simulink model "test_10gbe_out"  (Simulink 6.2)
settings: Solver=ode45  StartTime=0.0  StopTime=40000  RelTol=1e-3
libraries: xbsIndex_r3 x217, casper_library x8, xps_library x5
(part 1 of 2)
settings Model: LastModifiedBy=Jason Manley
settings DebuggingCC: SolverPrmCheckMsg=warning

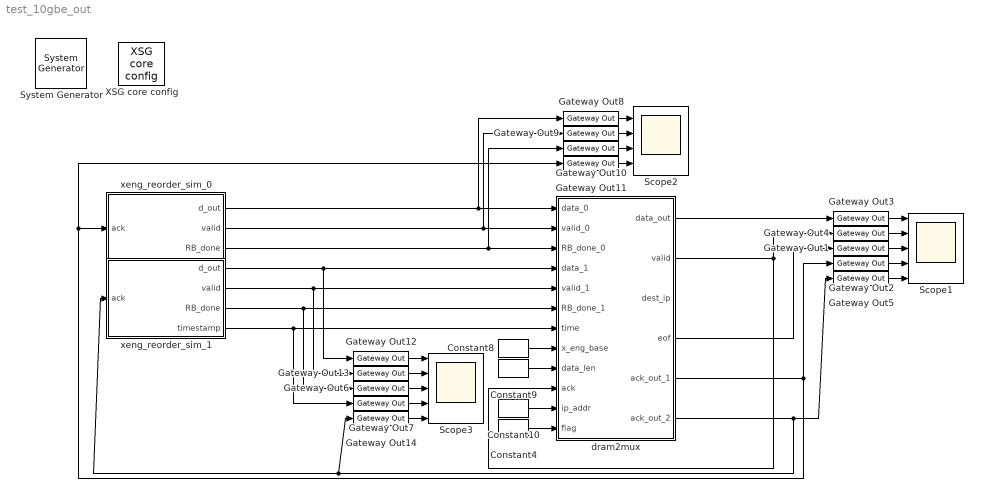
== system test_10gbe_out ==
  " System Generator" : xbsIndex_r3/ System Generator  Tag=genX  xilinxfamily=Virtex2  part=xc2v1000  speed=-4  package=bg575  synthesis_tool=XST  directory=./netlist  testbench=off  simulink_period=1  sysclk_period=100  incr_netlist=off  trim_vbits=Everywhere in SubSystem  dbl_ovrd=According to Block Masks  core_generation=According to Block Masks  run_coregen=off  deprecated_control=off  eval_field=0
      settings: AttributesFormatString=System\nGenerator
  Constant10 : xbsIndex_r3/Constant  const=1000  equ=P=C  arith_type=Unsigned  n_bits=32  bin_pt=0  opselect=C  inp2=PCIN>>17  opr=+  inp1=P  carry=CIN  iostate=0  explicit_period=on  period=1  dbl_ovrd=off
  Constant4 : xbsIndex_r3/Constant  const=0  equ=P=C  arith_type=Unsigned  n_bits=32  bin_pt=0  opselect=C  inp2=PCIN>>17  opr=+  inp1=P  carry=CIN  iostate=0  explicit_period=on  period=1  dbl_ovrd=off
  Constant8 : xbsIndex_r3/Constant  const=8  equ=P=C  arith_type=Unsigned  n_bits=16  bin_pt=0  opselect=C  inp2=PCIN>>17  opr=+  inp1=P  carry=CIN  iostate=0  explicit_period=on  period=1  dbl_ovrd=off
  Constant9 : xbsIndex_r3/Constant  const=180  equ=P=C  arith_type=Unsigned  n_bits=32  bin_pt=0  opselect=C  inp2=PCIN>>17  opr=+  inp1=P  carry=CIN  iostate=0  explicit_period=on  period=1  dbl_ovrd=off
  Gateway Out{1..14} (14 alike) : xbsIndex_r3/Gateway Out  output_type=Double  nbits=8  bin_pt=6  arith_type=Boolean  quantization=Truncate  overflow=Wrap  hdl_port=on  timing_constraint=None  locs_specified=off  LOCs={}  needs_fixed_name=off  show_param=off
      settings: xl_area=[0, 0, 0, 0, 0, 0, 0]
  Scope1 : Scope  NumInputPorts=5
      settings: YMin=432~-1~-1~-1~0  YMax=432~1~1~1~1  SaveName=ScopeData2
  Scope2 : Scope  NumInputPorts=4
      settings: YMin=0~0.95~0.95~-1  YMax=1~1.05~1.05~1
  Scope3 : Scope  NumInputPorts=5
      settings: YMin=10600~1~-1~-1~0  YMax=12200~1~1~1~1
  XSG core config : xps_library/XSG core config  Tag=xps:xsg  hw_sys=BEE2_usr  ibob_linux=off  clk_src=sys_clk2x  gpio_clk_io_group=iBOB:sma  gpio_clk_bit_index=0  clk_rate=205  sample_period=1  synthesis_tool=XST  mpc_type=powerpc405
  dram2mux : Subsystem  mask{payload_len=180}
      mask prompts: payload_len "Payload length"
  xeng_reorder_sim_0 : Subsystem
  xeng_reorder_sim_1 : Subsystem
  wires:
  dram2mux/5(ack_out_1) -> Gateway Out2/1, Gateway Out11/1, xeng_reorder_sim_0/1(ack)
  dram2mux/6(ack_out_2) -> Gateway Out5/1, Gateway Out14/1, xeng_reorder_sim_1/1(ack)
  Constant4/1 -> dram2mux/12(flag)
  Constant9/1 -> dram2mux/9(data_len)
  Constant10/1 -> dram2mux/11(ip_addr)
  dram2mux/2(valid) -> dram2mux/10(ack), Gateway Out4/1
  Gateway Out8/1 -> Scope2/1
  Gateway Out9/1 -> Scope2/2
  Gateway Out10/1 -> Scope2/3
  Gateway Out11/1 -> Scope2/4
  Gateway Out3/1 -> Scope1/1
  Gateway Out4/1 -> Scope1/2
  Gateway Out1/1 -> Scope1/3
  Gateway Out2/1 -> Scope1/4
  dram2mux/1(data_out) -> Gateway Out3/1
  dram2mux/4(eof) -> Gateway Out1/1
  Gateway Out5/1 -> Scope1/5
  xeng_reorder_sim_0/1(d_out) -> dram2mux/1(data_0), Gateway Out8/1
  xeng_reorder_sim_0/2(valid) -> dram2mux/2(valid_0), Gateway Out9/1
  Constant8/1 -> dram2mux/8(x_eng_base)
  xeng_reorder_sim_0/3(RB_done) -> dram2mux/3(RB_done_0), Gateway Out10/1
  xeng_reorder_sim_1/1(d_out) -> dram2mux/4(data_1), Gateway Out12/1
  xeng_reorder_sim_1/2(valid) -> dram2mux/5(valid_1), Gateway Out13/1
  xeng_reorder_sim_1/3(RB_done) -> dram2mux/6(RB_done_1), Gateway Out6/1
  xeng_reorder_sim_1/4(timestamp) -> dram2mux/7(time), Gateway Out7/1
  Gateway Out12/1 -> Scope3/1
  Gateway Out13/1 -> Scope3/2
  Gateway Out6/1 -> Scope3/3
  Gateway Out7/1 -> Scope3/4
  Gateway Out14/1 -> Scope3/5

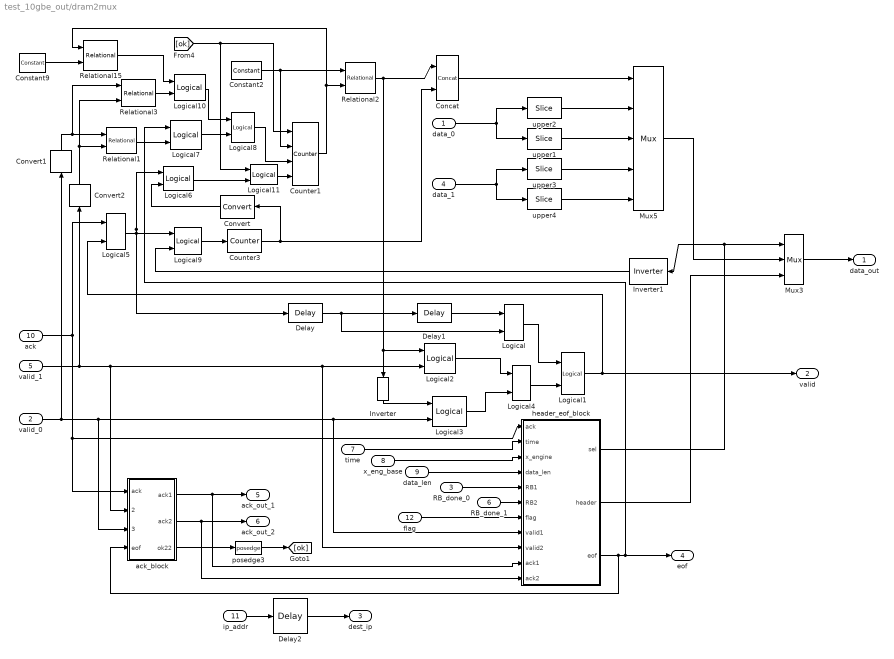
== system test_10gbe_out/dram2mux ==
  data_0 : Inport  Port=1  LatchInput=off
  valid_0 : Inport  Port=2  LatchInput=off
  RB_done_0 : Inport  Port=3  LatchInput=off
  data_1 : Inport  Port=4  LatchInput=off
  valid_1 : Inport  Port=5  LatchInput=off
  RB_done_1 : Inport  Port=6  LatchInput=off
  time : Inport  Port=7  LatchInput=off
  x_eng_base : Inport  Port=8  LatchInput=off
  data_len : Inport  Port=9  LatchInput=off
  ack : Inport  Port=10  LatchInput=off
  ip_addr : Inport  Port=11  LatchInput=off
  flag : Inport  Port=12  LatchInput=off
  Concat : xbsIndex_r3/Concat  num_inputs=2  explicit_period=off  period=1  dbl_ovrd=off
  Constant2 : xbsIndex_r3/Constant  const=payload_len/2  equ=P=C  arith_type=Unsigned  n_bits=16  bin_pt=0  opselect=C  inp2=PCIN>>17  opr=+  inp1=P  carry=CIN  iostate=0  explicit_period=on  period=1  dbl_ovrd=off
  Constant9 : xbsIndex_r3/Constant  const=payload_len  equ=P=C  arith_type=Unsigned  n_bits=8  bin_pt=0  opselect=C  inp2=PCIN>>17  opr=+  inp1=P  carry=CIN  iostate=0  explicit_period=on  period=1  dbl_ovrd=off
  Convert : xbsIndex_r3/Convert  Orientation=left  arith_type=Boolean  n_bits=8  bin_pt=6  quantization=Truncate  overflow=Wrap  latency=0  explicit_period=off  period=1  dbl_ovrd=off  show_param=off  inserted_by_tool=off  pipeline=off
      settings: xl_area=[0, 0, 0, 0, 0, 0, 0]
  Convert1 : xbsIndex_r3/Convert  Orientation=up  arith_type=Unsigned  n_bits=1  bin_pt=0  quantization=Truncate  overflow=Wrap  latency=0  explicit_period=off  period=1  dbl_ovrd=off  show_param=off  inserted_by_tool=off  pipeline=off
      settings: xl_area=[0, 0, 0, 0, 0, 0, 0]
  Convert2 : xbsIndex_r3/Convert  Orientation=up  arith_type=Unsigned  n_bits=1  bin_pt=0  quantization=Truncate  overflow=Wrap  latency=0  explicit_period=off  period=1  dbl_ovrd=off  show_param=off  inserted_by_tool=off  pipeline=off
      settings: xl_area=[0, 0, 0, 0, 0, 0, 0]
  Counter1 : xbsIndex_r3/Counter  cnt_type=Free Running  n_bits=16  bin_pt=0  arith_type=Unsigned  start_count=0  cnt_to=180  cnt_by_val=1  operation=Up  explicit_period=on  period=1  load_pin=on  rst=on  en=on  dbl_ovrd=off  show_param=off  use_rpm=on  gen_core=off
      settings: xl_area=[0, 0, 0, 0, 0, 0, 0]
  Counter3 : xbsIndex_r3/Counter  cnt_type=Free Running  n_bits=1  bin_pt=0  arith_type=Unsigned  start_count=0  cnt_to=Inf  cnt_by_val=1  operation=Up  explicit_period=on  period=1  load_pin=off  rst=off  en=on  dbl_ovrd=off  show_param=off  use_rpm=on  gen_core=off
      settings: xl_area=[0, 0, 0, 0, 0, 0, 0]
  Delay : xbsIndex_r3/Delay  latency=1  reg_retiming=off  explicit_period=on  period=1  en=off  accept_only_valid=off  init_zero=on  dbl_ovrd=off  show_param=off
      settings: xl_area=[0, 0, 0, 0, 0, 0, 0]
  Delay1 : xbsIndex_r3/Delay  latency=1  reg_retiming=off  explicit_period=on  period=1  en=off  accept_only_valid=off  init_zero=on  dbl_ovrd=off  show_param=off
      settings: xl_area=[0, 0, 0, 0, 0, 0, 0]
  Delay2 : xbsIndex_r3/Delay  latency=2  reg_retiming=off  explicit_period=off  period=1  en=off  accept_only_valid=off  init_zero=on  dbl_ovrd=off  show_param=off
      settings: xl_area=[0, 0, 0, 0, 0, 0, 0]
  Inverter : xbsIndex_r3/Inverter  Orientation=down  latency=0  explicit_period=off  period=1  en=off  dbl_ovrd=off  show_param=off
      settings: xl_area=[0, 0, 0, 0, 0, 0, 0]
  Inverter1 : xbsIndex_r3/Inverter  Orientation=left  latency=0  explicit_period=off  period=1  en=off  dbl_ovrd=off  show_param=off
      settings: xl_area=[0, 0, 0, 0, 0, 0, 0]
  Logical : xbsIndex_r3/Logical  logical_function=NOR  inputs=2  precision=Full  arith_type=Unsigned  n_bits=8  bin_pt=2  align_bp=on  latency=0  explicit_period=off  period=1  en=off  dbl_ovrd=off  show_param=off
      settings: xl_area=[0, 0, 0, 0, 0, 0, 0]
  Logical{1..3,5..7,10} (7 alike) : xbsIndex_r3/Logical  logical_function=AND  inputs=2  precision=Full  arith_type=Unsigned  n_bits=8  bin_pt=2  align_bp=off  latency=0  explicit_period=off  period=1  en=off  dbl_ovrd=off  show_param=off
      settings: xl_area=[0, 0, 0, 0, 0, 0, 0]
  Logical11 : xbsIndex_r3/Logical  logical_function=OR  inputs=2  precision=Full  arith_type=Unsigned  n_bits=8  bin_pt=2  align_bp=off  latency=0  explicit_period=off  period=1  en=off  dbl_ovrd=off  show_param=off
      settings: xl_area=[0, 0, 0, 0, 0, 0, 0]
  Logical4 : xbsIndex_r3/Logical  logical_function=OR  inputs=2  precision=Full  arith_type=Unsigned  n_bits=8  bin_pt=2  align_bp=on  latency=2  explicit_period=off  period=1  en=off  dbl_ovrd=off  show_param=off
      settings: xl_area=[0, 0, 0, 0, 0, 0, 0]
  Logical8 : xbsIndex_r3/Logical  logical_function=OR  inputs=2  precision=Full  arith_type=Unsigned  n_bits=8  bin_pt=2  align_bp=off  latency=0  explicit_period=off  period=1  en=off  dbl_ovrd=off  show_param=off
      settings: xl_area=[0, 0, 0, 0, 0, 0, 0]
  Logical9 : xbsIndex_r3/Logical  logical_function=AND  inputs=2  precision=Full  arith_type=Unsigned  n_bits=8  bin_pt=2  align_bp=on  latency=0  explicit_period=off  period=1  en=off  dbl_ovrd=off  show_param=off
      settings: xl_area=[0, 0, 0, 0, 0, 0, 0]
  Mux3 : xbsIndex_r3/Mux  inputs=2  precision=Full  arith_type="Signed  (2's comp)"  n_bits=8  bin_pt=2  quantization=Truncate  overflow=Wrap  latency=0  explicit_period=off  period=1  en=off  dbl_ovrd=off  show_param=off  mux_type=off  use_rpm=off  gen_core=off
      settings: xl_area=[0, 0, 0, 0, 0, 0, 0]
  Mux5 : xbsIndex_r3/Mux  inputs=4  precision=Full  arith_type="Signed  (2's comp)"  n_bits=8  bin_pt=2  quantization=Truncate  overflow=Wrap  latency=2  explicit_period=on  period=1  en=off  dbl_ovrd=off  show_param=off  mux_type=off  use_rpm=off  gen_core=off
      settings: xl_area=[0, 0, 0, 0, 0, 0, 0]
  Relational1 : xbsIndex_r3/Relational  mode=a>b  latency=0  explicit_period=off  period=1  en=off  dbl_ovrd=off  show_param=off
      settings: xl_area=[0, 0, 0, 0, 0, 0, 0]
  Relational15 : xbsIndex_r3/Relational  mode=a=b  latency=1  explicit_period=off  period=1  en=off  dbl_ovrd=off  show_param=off
      settings: xl_area=[0, 0, 0, 0, 0, 0, 0]
  Relational2 : xbsIndex_r3/Relational  mode=a<=b  latency=0  explicit_period=off  period=1  en=off  dbl_ovrd=off  show_param=off
      settings: xl_area=[0, 0, 0, 0, 0, 0, 0]
  Relational3 : xbsIndex_r3/Relational  mode=a>b  latency=0  explicit_period=off  period=1  en=off  dbl_ovrd=off  show_param=off
      settings: xl_area=[0, 0, 0, 0, 0, 0, 0]
  ack_block : Subsystem
  header_eof_block : Subsystem
  posedge3 : casper_library/Misc/posedge  Tag=Rising Edge Detector
  upper1 : xbsIndex_r3/Slice  mode=Lower Bit Location + Width  nbits=64  bit1=0  base1=MSB of Input  bit0=0  base0=LSB of Input  boolean_output=off  explicit_period=off  period=1  dbl_ovrd=off
  upper2 : xbsIndex_r3/Slice  mode=Upper Bit Location + Width  nbits=64  bit1=0  base1=MSB of Input  bit0=0  base0=LSB of Input  boolean_output=off  explicit_period=off  period=1  dbl_ovrd=off
  upper3 : xbsIndex_r3/Slice  mode=Upper Bit Location + Width  nbits=64  bit1=0  base1=MSB of Input  bit0=0  base0=LSB of Input  boolean_output=off  explicit_period=off  period=1  dbl_ovrd=off
  upper4 : xbsIndex_r3/Slice  mode=Lower Bit Location + Width  nbits=64  bit1=0  base1=MSB of Input  bit0=0  base0=LSB of Input  boolean_output=off  explicit_period=off  period=1  dbl_ovrd=off
  data_out : Outport
  valid : Outport  Port=2
  dest_ip : Outport  Port=3
  eof : Outport  Port=4
  ack_out_1 : Outport  Port=5
  ack_out_2 : Outport  Port=6
  wires:
  ack_block/2(ack2) -> ack_out_2/1, header_eof_block/11(ack2)
  ack_block/1(ack1) -> ack_out_1/1, header_eof_block/10(ack1)
  Inverter1/1 -> Logical9/2
  Mux5/1 -> Mux3/2
  data_len/1 -> header_eof_block/4(data_len)
  Delay2/1 -> dest_ip/1
  ip_addr/1 -> Delay2/1
  Mux3/1 -> data_out/1
  header_eof_block/2(header) -> Mux3/3
  x_eng_base/1 -> header_eof_block/3(x_engine)
  time/1 -> header_eof_block/2(time)
  Logical5/1 -> Logical6/1, Logical9/1, Delay/1
  Logical4/1 -> Logical1/2
  Logical3/1 -> Logical4/2
  Logical2/1 -> Logical4/1
  valid_1/1 -> ack_block/2(valid2), Logical2/2, header_eof_block/9(valid2), Convert2/1
  valid_0/1 -> ack_block/3(valid1), Logical3/2, header_eof_block/8(valid1), Convert1/1
  Logical1/1 -> valid/1, Logical5/2
  Logical/1 -> Logical1/1
  Delay1/1 -> Logical/1
  Delay/1 -> Delay1/1, Logical/2
  ack/1 -> Logical5/1, header_eof_block/1(ack), ack_block/1(ack)
  Concat/1 -> Mux5/1
  Relational2/1 -> Inverter/1, Logical2/1, Concat/1
  Constant2/1 -> Relational2/1, Counter1/2
  data_1/1 -> upper3/1, upper4/1
  data_0/1 -> upper2/1, upper1/1
  upper4/1 -> Mux5/5
  upper3/1 -> Mux5/4
  upper1/1 -> Mux5/3
  upper2/1 -> Mux5/2
  Inverter/1 -> Logical3/1
  Convert/1 -> Logical6/2
  Counter3/1 -> Convert/1, Concat/2
  Logical9/1 -> Counter3/1
  Constant9/1 -> Relational15/2
  header_eof_block/1(sel) -> Inverter1/1, Mux3/1
  header_eof_block/3(eof) -> eof/1, Logical7/1, ack_block/4(eof)
  RB_done_0/1 -> header_eof_block/5(RB1)
  RB_done_1/1 -> header_eof_block/6(RB2)
  flag/1 -> header_eof_block/7(flag)
  Logical7/1 -> Logical8/2
  Relational1/1 -> Logical7/2
  Convert1/1 -> Relational1/1, Relational3/1
  Convert2/1 -> Relational1/2, Relational3/2
  Relational15/1 -> Logical10/1
  Relational3/1 -> Logical10/2
  Logical8/1 -> Counter1/3
  Logical6/1 -> Logical11/2
  Logical11/1 -> Counter1/4
  ack_block/3(ok22) -> posedge3/1
  posedge3/1 -> [ok]
  Logical10/1 -> Logical8/1
  Counter1/1 -> Relational2/2, Relational15/1
  [ok] -> Counter1/1, Logical11/1

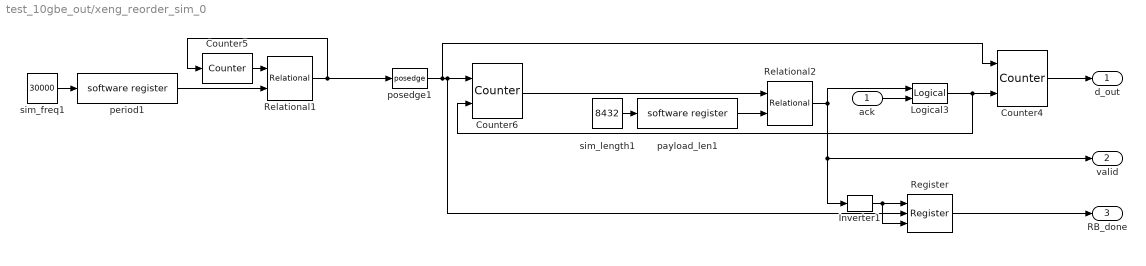
== system test_10gbe_out/xeng_reorder_sim_0 ==
  ack : Inport  Port=1  LatchInput=off
  Counter4 : xbsIndex_r3/Counter  cnt_type=Free Running  n_bits=64  bin_pt=0  arith_type=Unsigned  start_count=0  cnt_to=Inf  cnt_by_val=1  operation=Up  explicit_period=off  period=1  load_pin=off  rst=on  en=on  dbl_ovrd=off  show_param=off  use_rpm=off  gen_core=off
      settings: xl_area=[0, 0, 0, 0, 0, 0, 0]
  Counter5 : xbsIndex_r3/Counter  cnt_type=Free Running  n_bits=32  bin_pt=0  arith_type=Unsigned  start_count=1  cnt_to=Inf  cnt_by_val=1  operation=Up  explicit_period=on  period=1  load_pin=off  rst=on  en=off  dbl_ovrd=off  show_param=off  use_rpm=on  gen_core=off
      settings: xl_area=[0, 0, 0, 0, 0, 0, 0]
  Counter6 : xbsIndex_r3/Counter  cnt_type=Free Running  n_bits=32  bin_pt=0  arith_type=Unsigned  start_count=0  cnt_to=1023  cnt_by_val=1  operation=Up  explicit_period=on  period=1  load_pin=off  rst=on  en=on  dbl_ovrd=off  show_param=off  use_rpm=on  gen_core=off
      settings: xl_area=[0, 0, 0, 0, 0, 0, 0]
  Inverter1 : xbsIndex_r3/Inverter  latency=0  explicit_period=off  period=1  en=off  dbl_ovrd=off  show_param=off
      settings: xl_area=[0, 0, 0, 0, 0, 0, 0]
  Logical3 : xbsIndex_r3/Logical  logical_function=AND  inputs=2  precision=Full  arith_type=Unsigned  n_bits=8  bin_pt=2  align_bp=on  latency=0  explicit_period=off  period=1  en=off  dbl_ovrd=off  show_param=off
      settings: xl_area=[0, 0, 0, 0, 0, 0, 0]
  Register : xbsIndex_r3/Register  init=0  reg_only_valid=off  explicit_period=off  period=1  rst=on  en=on  out_en=off  dbl_ovrd=off  show_param=off
      settings: xl_area=[0, 0, 0, 0, 0, 0, 0]
  Relational1 : xbsIndex_r3/Relational  mode=a>=b  latency=0  explicit_period=on  period=1  en=off  dbl_ovrd=off  show_param=off
      settings: xl_area=[0, 0, 0, 0, 0, 0, 0]
  Relational2 : xbsIndex_r3/Relational  mode=a<b  latency=0  explicit_period=off  period=1  en=off  dbl_ovrd=off  show_param=off
      settings: xl_area=[0, 0, 0, 0, 0, 0, 0]
  payload_len1 : xps_library/software register  Tag=xps:sw_reg  io_dir=From Processor  arith_type=Unsigned  bitwidth=32  bin_pt=0  sample_period=1  gw_name=test_10gbe_out_xeng_reorder_sim_0_payload_len1_user_data_out
  period1 : xps_library/software register  Tag=xps:sw_reg  io_dir=From Processor  arith_type=Unsigned  bitwidth=32  bin_pt=0  sample_period=1  gw_name=test_10gbe_out_xeng_reorder_sim_0_period1_user_data_out
  posedge1 : casper_library/Misc/pulse_ext/posedge  Tag=Rising Edge Detector
  sim_freq1 : Constant  Value=30000
  sim_length1 : Constant  Value=8432
  d_out : Outport
  valid : Outport  Port=2
  RB_done : Outport  Port=3
  wires:
  Counter5/1 -> Relational1/1
  Relational1/1 -> Counter5/1, posedge1/1
  Counter4/1 -> d_out/1
  period1/1 -> Relational1/2
  sim_freq1/1 -> period1/1
  Relational2/1 -> Inverter1/1, valid/1, Logical3/1
  Counter6/1 -> Relational2/1
  posedge1/1 -> Counter4/1, Counter6/1, Register/2
  sim_length1/1 -> payload_len1/1
  Logical3/1 -> Counter4/2, Counter6/2
  payload_len1/1 -> Relational2/2
  Register/1 -> RB_done/1
  Inverter1/1 -> Register/1, Register/3
  ack/1 -> Logical3/2

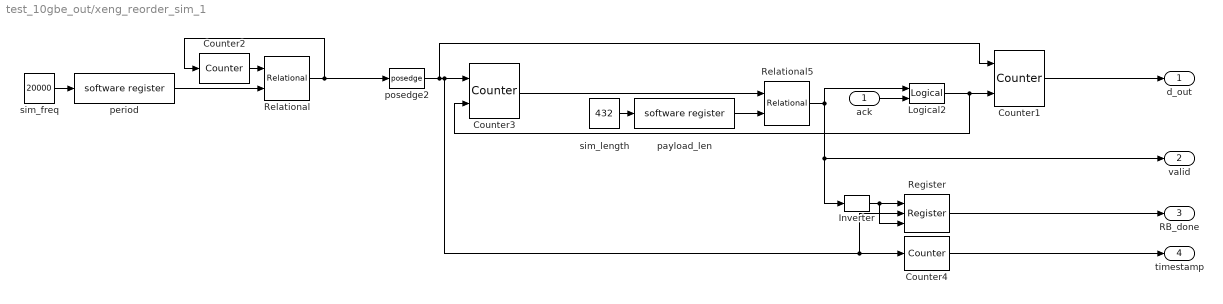
== system test_10gbe_out/xeng_reorder_sim_1 ==
  ack : Inport  Port=1  LatchInput=off
  Counter1 : xbsIndex_r3/Counter  cnt_type=Free Running  n_bits=64  bin_pt=0  arith_type=Unsigned  start_count=0  cnt_to=Inf  cnt_by_val=1  operation=Up  explicit_period=off  period=1  load_pin=off  rst=on  en=on  dbl_ovrd=off  show_param=off  use_rpm=off  gen_core=off
      settings: xl_area=[0, 0, 0, 0, 0, 0, 0]
  Counter2 : xbsIndex_r3/Counter  cnt_type=Free Running  n_bits=32  bin_pt=0  arith_type=Unsigned  start_count=1  cnt_to=Inf  cnt_by_val=1  operation=Up  explicit_period=on  period=1  load_pin=off  rst=on  en=off  dbl_ovrd=off  show_param=off  use_rpm=on  gen_core=off
      settings: xl_area=[0, 0, 0, 0, 0, 0, 0]
  Counter3 : xbsIndex_r3/Counter  cnt_type=Free Running  n_bits=32  bin_pt=0  arith_type=Unsigned  start_count=0  cnt_to=1023  cnt_by_val=1  operation=Up  explicit_period=on  period=1  load_pin=off  rst=on  en=on  dbl_ovrd=off  show_param=off  use_rpm=on  gen_core=off
      settings: xl_area=[0, 0, 0, 0, 0, 0, 0]
  Counter4 : xbsIndex_r3/Counter  cnt_type=Free Running  n_bits=64  bin_pt=0  arith_type=Unsigned  start_count=0  cnt_to=1023  cnt_by_val=1  operation=Up  explicit_period=on  period=1  load_pin=off  rst=off  en=on  dbl_ovrd=off  show_param=off  use_rpm=on  gen_core=off
      settings: xl_area=[0, 0, 0, 0, 0, 0, 0]
  Inverter : xbsIndex_r3/Inverter  latency=0  explicit_period=off  period=1  en=off  dbl_ovrd=off  show_param=off
      settings: xl_area=[0, 0, 0, 0, 0, 0, 0]
  Logical2 : xbsIndex_r3/Logical  logical_function=AND  inputs=2  precision=Full  arith_type=Unsigned  n_bits=8  bin_pt=2  align_bp=on  latency=0  explicit_period=off  period=1  en=off  dbl_ovrd=off  show_param=off
      settings: xl_area=[0, 0, 0, 0, 0, 0, 0]
  Register : xbsIndex_r3/Register  init=0  reg_only_valid=off  explicit_period=off  period=1  rst=on  en=on  out_en=off  dbl_ovrd=off  show_param=off
      settings: xl_area=[0, 0, 0, 0, 0, 0, 0]
  Relational : xbsIndex_r3/Relational  mode=a>=b  latency=0  explicit_period=on  period=1  en=off  dbl_ovrd=off  show_param=off
      settings: xl_area=[0, 0, 0, 0, 0, 0, 0]
  Relational5 : xbsIndex_r3/Relational  mode=a<b  latency=0  explicit_period=off  period=1  en=off  dbl_ovrd=off  show_param=off
      settings: xl_area=[0, 0, 0, 0, 0, 0, 0]
  payload_len : xps_library/software register  Tag=xps:sw_reg  io_dir=From Processor  arith_type=Unsigned  bitwidth=32  bin_pt=0  sample_period=1  gw_name=test_10gbe_out_xeng_reorder_sim_1_payload_len_user_data_out
  period : xps_library/software register  Tag=xps:sw_reg  io_dir=From Processor  arith_type=Unsigned  bitwidth=32  bin_pt=0  sample_period=1  gw_name=test_10gbe_out_xeng_reorder_sim_1_period_user_data_out
  posedge2 : casper_library/Misc/pulse_ext/posedge  Tag=Rising Edge Detector
  sim_freq : Constant  Value=20000
  sim_length : Constant  Value=432
  d_out : Outport
  valid : Outport  Port=2
  RB_done : Outport  Port=3
  timestamp : Outport  Port=4
  wires:
  Counter2/1 -> Relational/1
  Relational/1 -> Counter2/1, posedge2/1
  Counter1/1 -> d_out/1
  period/1 -> Relational/2
  sim_freq/1 -> period/1
  Relational5/1 -> Inverter/1, valid/1, Logical2/1
  Counter3/1 -> Relational5/1
  posedge2/1 -> Counter1/1, Counter3/1, Counter4/1, Register/2
  sim_length/1 -> payload_len/1
  Logical2/1 -> Counter1/2, Counter3/2
  payload_len/1 -> Relational5/2
  Register/1 -> RB_done/1
  Counter4/1 -> timestamp/1
  Inverter/1 -> Register/1, Register/3
  ack/1 -> Logical2/2

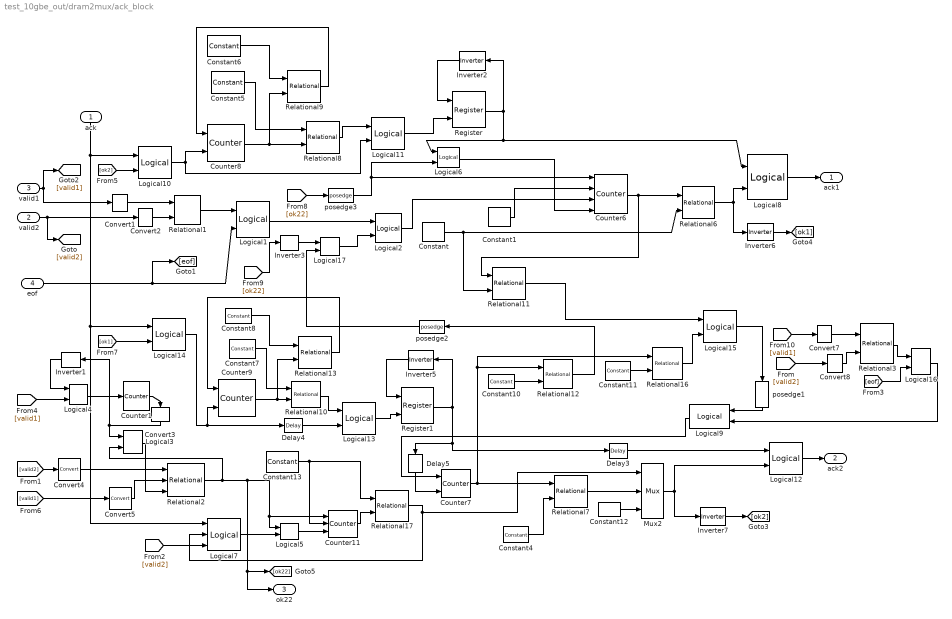
== system test_10gbe_out/dram2mux/ack_block ==
  ack : Inport  Orientation=down  Port=1  LatchInput=off
  valid2 : Inport  Port=2  LatchInput=off
  valid1 : Inport  Port=3  LatchInput=off
  eof : Inport  Port=4  LatchInput=off
  Constant : xbsIndex_r3/Constant  const=payload_len*3/2 -1  equ=P=C  arith_type=Unsigned  n_bits=10  bin_pt=0  opselect=C  inp2=PCIN>>17  opr=+  inp1=P  carry=CIN  iostate=0  explicit_period=on  period=1  dbl_ovrd=off
  Constant1 : xbsIndex_r3/Constant  const=payload_len*3/2  equ=P=C  arith_type=Unsigned  n_bits=10  bin_pt=0  opselect=C  inp2=PCIN>>17  opr=+  inp1=P  carry=CIN  iostate=0  explicit_period=on  period=1  dbl_ovrd=off
  Constant10 : xbsIndex_r3/Constant  const=payload_len*3/2 -1  equ=P=C  arith_type=Unsigned  n_bits=9  bin_pt=0  opselect=C  inp2=PCIN>>17  opr=+  inp1=P  carry=CIN  iostate=0  explicit_period=on  period=1  dbl_ovrd=off
  Constant11 : xbsIndex_r3/Constant  const=payload_len*3/2+1  equ=P=C  arith_type=Unsigned  n_bits=9  bin_pt=0  opselect=C  inp2=PCIN>>17  opr=+  inp1=P  carry=CIN  iostate=0  explicit_period=on  period=1  dbl_ovrd=off
  Constant12 : xbsIndex_r3/Constant  const=0  equ=P=C  arith_type=Boolean  n_bits=1  bin_pt=0  opselect=C  inp2=PCIN>>17  opr=+  inp1=P  carry=CIN  iostate=0  explicit_period=on  period=1  dbl_ovrd=off
  Constant13 : xbsIndex_r3/Constant  const=payload_len+3  equ=P=C  arith_type=Unsigned  n_bits=10  bin_pt=0  opselect=C  inp2=PCIN>>17  opr=+  inp1=P  carry=CIN  iostate=0  explicit_period=on  period=1  dbl_ovrd=off
  Constant4 : xbsIndex_r3/Constant  const=payload_len*3/2-1  equ=P=C  arith_type=Unsigned  n_bits=9  bin_pt=0  opselect=C  inp2=PCIN>>17  opr=+  inp1=P  carry=CIN  iostate=0  explicit_period=on  period=1  dbl_ovrd=off
  Constant5 : xbsIndex_r3/Constant  const=3  equ=P=C  arith_type=Unsigned  n_bits=2  bin_pt=0  opselect=C  inp2=PCIN>>17  opr=+  inp1=P  carry=CIN  iostate=0  explicit_period=on  period=1  dbl_ovrd=off
  Constant6 : xbsIndex_r3/Constant  const=payload_len+3  equ=P=C  arith_type=Unsigned  n_bits=8  bin_pt=0  opselect=C  inp2=PCIN>>17  opr=+  inp1=P  carry=CIN  iostate=0  explicit_period=on  period=1  dbl_ovrd=off
  Constant7 : xbsIndex_r3/Constant  const=3  equ=P=C  arith_type=Unsigned  n_bits=2  bin_pt=0  opselect=C  inp2=PCIN>>17  opr=+  inp1=P  carry=CIN  iostate=0  explicit_period=on  period=1  dbl_ovrd=off
  Constant8 : xbsIndex_r3/Constant  const=payload_len+3  equ=P=C  arith_type=Unsigned  n_bits=8  bin_pt=0  opselect=C  inp2=PCIN>>17  opr=+  inp1=P  carry=CIN  iostate=0  explicit_period=on  period=1  dbl_ovrd=off
  Convert{1..2,4..5,7..8} (6 alike) : xbsIndex_r3/Convert  arith_type=Unsigned  n_bits=1  bin_pt=0  quantization=Truncate  overflow=Wrap  latency=0  explicit_period=off  period=1  dbl_ovrd=off  show_param=off  inserted_by_tool=off  pipeline=off
      settings: xl_area=[0, 0, 0, 0, 0, 0, 0]
  Convert3 : xbsIndex_r3/Convert  Orientation=down  arith_type=Boolean  n_bits=1  bin_pt=0  quantization=Truncate  overflow=Wrap  latency=0  explicit_period=off  period=1  dbl_ovrd=off  show_param=off  inserted_by_tool=off  pipeline=off
      settings: xl_area=[0, 0, 0, 0, 0, 0, 0]
  Counter1 : xbsIndex_r3/Counter  cnt_type=Count Limited  n_bits=1  bin_pt=0  arith_type=Unsigned  start_count=0  cnt_to=1  cnt_by_val=1  operation=Up  explicit_period=on  period=1  load_pin=off  rst=off  en=on  dbl_ovrd=off  show_param=off  use_rpm=on  gen_core=off
      settings: xl_area=[0, 0, 0, 0, 0, 0, 0]
  Counter11 : xbsIndex_r3/Counter  cnt_type=Free Running  n_bits=10  bin_pt=0  arith_type=Unsigned  start_count=0  cnt_to=Inf  cnt_by_val=1  operation=Up  explicit_period=on  period=1  load_pin=on  rst=off  en=on  dbl_ovrd=off  show_param=off  use_rpm=on  gen_core=off
      settings: xl_area=[0, 0, 0, 0, 0, 0, 0]
  Counter6 : xbsIndex_r3/Counter  cnt_type=Free Running  n_bits=10  bin_pt=0  arith_type=Unsigned  start_count=0  cnt_to=Inf  cnt_by_val=1  operation=Up  explicit_period=on  period=1  load_pin=on  rst=on  en=on  dbl_ovrd=off  show_param=off  use_rpm=on  gen_core=off
      settings: xl_area=[0, 0, 0, 0, 0, 0, 0]
  Counter7 : xbsIndex_r3/Counter  cnt_type=Free Running  n_bits=10  bin_pt=0  arith_type=Unsigned  start_count=0  cnt_to=Inf  cnt_by_val=1  operation=Up  explicit_period=on  period=1  load_pin=off  rst=on  en=on  dbl_ovrd=off  show_param=off  use_rpm=on  gen_core=off
      settings: xl_area=[0, 0, 0, 0, 0, 0, 0]
  Counter8 : xbsIndex_r3/Counter  cnt_type=Free Running  n_bits=8  bin_pt=0  arith_type=Unsigned  start_count=0  cnt_to=Inf  cnt_by_val=1  operation=Up  explicit_period=on  period=1  load_pin=off  rst=on  en=on  dbl_ovrd=off  show_param=off  use_rpm=on  gen_core=off
      settings: xl_area=[0, 0, 0, 0, 0, 0, 0]
  Counter9 : xbsIndex_r3/Counter  cnt_type=Free Running  n_bits=8  bin_pt=0  arith_type=Unsigned  start_count=0  cnt_to=Inf  cnt_by_val=1  operation=Up  explicit_period=on  period=1  load_pin=off  rst=on  en=on  dbl_ovrd=off  show_param=off  use_rpm=on  gen_core=off
      settings: xl_area=[0, 0, 0, 0, 0, 0, 0]
  Delay3 : xbsIndex_r3/Delay  latency=1  reg_retiming=off  explicit_period=on  period=1  en=off  accept_only_valid=off  init_zero=on  dbl_ovrd=off  show_param=off
      settings: xl_area=[0, 0, 0, 0, 0, 0, 0]
  Delay4 : xbsIndex_r3/Delay  latency=2  reg_retiming=off  explicit_period=on  period=1  en=off  accept_only_valid=off  init_zero=on  dbl_ovrd=off  show_param=off
      settings: xl_area=[0, 0, 0, 0, 0, 0, 0]
  Delay5 : xbsIndex_r3/Delay  Orientation=down  latency=1  reg_retiming=off  explicit_period=on  period=1  en=off  accept_only_valid=off  init_zero=on  dbl_ovrd=off  show_param=off
      settings: xl_area=[0, 0, 0, 0, 0, 0, 0]
  Inverter1 : xbsIndex_r3/Inverter  Orientation=left  latency=0  explicit_period=off  period=1  en=off  dbl_ovrd=off  show_param=off
      settings: xl_area=[0, 0, 0, 0, 0, 0, 0]
  Inverter2 : xbsIndex_r3/Inverter  Orientation=left  latency=0  explicit_period=off  period=1  en=off  dbl_ovrd=off  show_param=off
      settings: xl_area=[0, 0, 0, 0, 0, 0, 0]
  Inverter3 : xbsIndex_r3/Inverter  latency=0  explicit_period=off  period=1  en=off  dbl_ovrd=off  show_param=off
      settings: xl_area=[0, 0, 0, 0, 0, 0, 0]
  Inverter5 : xbsIndex_r3/Inverter  Orientation=left  latency=0  explicit_period=off  period=1  en=off  dbl_ovrd=off  show_param=off
      settings: xl_area=[0, 0, 0, 0, 0, 0, 0]
  Inverter6 : xbsIndex_r3/Inverter  latency=0  explicit_period=off  period=1  en=off  dbl_ovrd=off  show_param=off
      settings: xl_area=[0, 0, 0, 0, 0, 0, 0]
  Inverter7 : xbsIndex_r3/Inverter  latency=0  explicit_period=off  period=1  en=off  dbl_ovrd=off  show_param=off
      settings: xl_area=[0, 0, 0, 0, 0, 0, 0]
  Logical{1,4,10..11,13..14,16..17} (8 alike) : xbsIndex_r3/Logical  logical_function=AND  inputs=2  precision=Full  arith_type=Unsigned  n_bits=8  bin_pt=2  align_bp=on  latency=0  explicit_period=off  period=1  en=off  dbl_ovrd=off  show_param=off
      settings: xl_area=[0, 0, 0, 0, 0, 0, 0]
  Logical12 : xbsIndex_r3/Logical  logical_function=AND  inputs=2  precision=Full  arith_type=Unsigned  n_bits=8  bin_pt=2  align_bp=on  latency=2  explicit_period=on  period=1  en=off  dbl_ovrd=off  show_param=off
      settings: xl_area=[0, 0, 0, 0, 0, 0, 0]
  Logical15 : xbsIndex_r3/Logical  logical_function=OR  inputs=2  precision=Full  arith_type=Unsigned  n_bits=8  bin_pt=2  align_bp=on  latency=0  explicit_period=off  period=1  en=off  dbl_ovrd=off  show_param=off
      settings: xl_area=[0, 0, 0, 0, 0, 0, 0]
  Logical2 : xbsIndex_r3/Logical  logical_function=OR  inputs=2  precision=Full  arith_type=Unsigned  n_bits=8  bin_pt=2  align_bp=off  latency=0  explicit_period=off  period=1  en=off  dbl_ovrd=off  show_param=off
      settings: xl_area=[0, 0, 0, 0, 0, 0, 0]
  Logical3 : xbsIndex_r3/Logical  logical_function=NOR  inputs=2  precision=Full  arith_type=Unsigned  n_bits=8  bin_pt=2  align_bp=off  latency=0  explicit_period=on  period=1  en=off  dbl_ovrd=off  show_param=off
      settings: xl_area=[0, 0, 0, 0, 0, 0, 0]
  Logical5 : xbsIndex_r3/Logical  logical_function=OR  inputs=2  precision=Full  arith_type=Unsigned  n_bits=8  bin_pt=2  align_bp=off  latency=0  explicit_period=off  period=1  en=off  dbl_ovrd=off  show_param=off
      settings: xl_area=[0, 0, 0, 0, 0, 0, 0]
  Logical6 : xbsIndex_r3/Logical  logical_function=OR  inputs=2  precision=Full  arith_type=Unsigned  n_bits=8  bin_pt=2  align_bp=off  latency=0  explicit_period=off  period=1  en=off  dbl_ovrd=off  show_param=off
      settings: xl_area=[0, 0, 0, 0, 0, 0, 0]
  Logical7 : xbsIndex_r3/Logical  logical_function=AND  inputs=3  precision=Full  arith_type=Unsigned  n_bits=8  bin_pt=2  align_bp=on  latency=0  explicit_period=off  period=1  en=off  dbl_ovrd=off  show_param=off
      settings: xl_area=[0, 0, 0, 0, 0, 0, 0]
  Logical8 : xbsIndex_r3/Logical  logical_function=AND  inputs=2  precision=Full  arith_type=Unsigned  n_bits=8  bin_pt=2  align_bp=on  latency=2  explicit_period=on  period=1  en=off  dbl_ovrd=off  show_param=off
      settings: xl_area=[0, 0, 0, 0, 0, 0, 0]
  Logical9 : xbsIndex_r3/Logical  Orientation=left  logical_function=OR  inputs=2  precision=Full  arith_type=Unsigned  n_bits=8  bin_pt=2  align_bp=off  latency=0  explicit_period=off  period=1  en=off  dbl_ovrd=off  show_param=off
      settings: xl_area=[0, 0, 0, 0, 0, 0, 0]
  Mux2 : xbsIndex_r3/Mux  inputs=2  precision=Full  arith_type="Signed  (2's comp)"  n_bits=8  bin_pt=2  quantization=Truncate  overflow=Wrap  latency=0  explicit_period=off  period=1  en=off  dbl_ovrd=off  show_param=off  mux_type=off  use_rpm=off  gen_core=off
      settings: xl_area=[0, 0, 0, 0, 0, 0, 0]
  Register : xbsIndex_r3/Register  init=0  reg_only_valid=off  explicit_period=on  period=1  rst=off  en=on  out_en=off  dbl_ovrd=off  show_param=off
      settings: xl_area=[0, 0, 0, 0, 0, 0, 0]
  Register1 : xbsIndex_r3/Register  init=0  reg_only_valid=off  explicit_period=on  period=1  rst=off  en=on  out_en=off  dbl_ovrd=off  show_param=off
      settings: xl_area=[0, 0, 0, 0, 0, 0, 0]
  Relational1 : xbsIndex_r3/Relational  mode=a>b  latency=0  explicit_period=off  period=1  en=off  dbl_ovrd=off  show_param=off
      settings: xl_area=[0, 0, 0, 0, 0, 0, 0]
  Relational{6..8,10} (4 alike) : xbsIndex_r3/Relational  mode=a<=b  latency=0  explicit_period=off  period=1  en=off  dbl_ovrd=off  show_param=off
      settings: xl_area=[0, 0, 0, 0, 0, 0, 0]
  Relational11 : xbsIndex_r3/Relational  mode=a=b  latency=0  explicit_period=on  period=1  en=off  dbl_ovrd=off  show_param=off
      settings: xl_area=[0, 0, 0, 0, 0, 0, 0]
  Relational{9,12..13,16} (4 alike) : xbsIndex_r3/Relational  mode=a=b  latency=0  explicit_period=off  period=1  en=off  dbl_ovrd=off  show_param=off
      settings: xl_area=[0, 0, 0, 0, 0, 0, 0]
  Relational17 : xbsIndex_r3/Relational  mode=a>b  latency=0  explicit_period=off  period=1  en=off  dbl_ovrd=off  show_param=off
      settings: xl_area=[0, 0, 0, 0, 0, 0, 0]
  Relational2 : xbsIndex_r3/Relational  mode=a>b  latency=1  explicit_period=off  period=1  en=on  dbl_ovrd=off  show_param=off
      settings: xl_area=[0, 0, 0, 0, 0, 0, 0]
  Relational3 : xbsIndex_r3/Relational  mode=a<b  latency=0  explicit_period=off  period=1  en=off  dbl_ovrd=off  show_param=off
      settings: xl_area=[0, 0, 0, 0, 0, 0, 0]
  posedge1 : casper_library/Misc/posedge  Tag=Rising Edge Detector  Orientation=down
  posedge2 : casper_library/Misc/posedge  Tag=Rising Edge Detector  Orientation=left
  posedge3 : casper_library/Misc/posedge  Tag=Rising Edge Detector
  ack1 : Outport
  ack2 : Outport  Port=2
  ok22 : Outport  Port=3
  wires:
  Logical14/1 -> Counter9/2, Delay4/1
  Logical10/1 -> Counter8/2, Logical11/2
  Logical13/1 -> Register1/2
  Constant4/1 -> Relational7/2
  Counter7/1 -> Relational7/1, Relational12/1, Relational16/1
  Inverter5/1 -> Register1/1
  Register1/1 -> Delay3/1, Delay5/1, Inverter5/1
  Relational9/1 -> Counter8/1
  Constant6/1 -> Relational9/1
  Constant5/1 -> Relational8/1
  Counter8/1 -> Relational8/2, Relational9/2
  Relational6/1 -> Logical8/2, Inverter6/1
  Constant/1 -> Relational6/2, Relational11/2
  Counter6/1 -> Relational11/1, Relational6/1
  Inverter2/1 -> Register/1
  Register/1 -> Logical8/1, Logical6/1, Inverter2/1
  Relational8/1 -> Logical11/1
  Logical11/1 -> Register/2
  Relational13/1 -> Counter9/1
  Constant8/1 -> Relational13/1
  Constant7/1 -> Relational10/1
  Counter9/1 -> Relational10/2, Relational13/2
  Relational10/1 -> Logical13/1
  Delay4/1 -> Logical13/2
  Relational12/1 -> posedge2/1
  Relational11/1 -> Logical15/1
  Constant11/1 -> Relational16/2
  Relational16/1 -> Logical15/2
  Logical15/1 -> posedge1/1
  Constant10/1 -> Relational12/2
  Delay3/1 -> Logical12/1
  Mux2/1 -> Logical12/2, Inverter7/1
  Relational7/1 -> Mux2/2
  Constant12/1 -> Mux2/3
  Constant13/1 -> Relational17/1, Counter11/2
  Counter11/1 -> Relational17/2
  Relational17/1 -> Mux2/1, Logical7/2
  Delay5/1 -> Counter7/2
  ack/1 -> Logical10/1, Logical14/1, Logical7/1
  Logical8/1 -> ack1/1
  Logical12/1 -> ack2/1
  valid2/1 -> [valid2], Convert2/1
  valid1/1 -> [valid1], Convert1/1
  Relational1/1 -> Logical1/1
  Logical1/1 -> Logical2/1
  Convert1/1 -> Relational1/1
  Convert2/1 -> Relational1/2
  eof/1 -> Logical1/2, [eof]
  Relational2/1 -> Logical3/2, Counter11/1, Logical5/1, ok22/1, [ok22]
  Counter1/1 -> Convert3/1
  Logical3/1 -> Relational2/3
  Convert3/1 -> Logical3/1, Inverter1/1
  Convert4/1 -> Relational2/1
  Convert5/1 -> Relational2/2
  Logical4/1 -> Counter1/1
  Inverter1/1 -> Logical4/1
  Logical7/1 -> Logical5/2
  Logical5/1 -> Counter11/3
  Logical2/1 -> Counter6/3
  posedge3/1 -> Counter6/1, Logical6/2
  Constant1/1 -> Counter6/2
  posedge1/1 -> Logical9/1
  Logical9/1 -> Counter7/1
  Convert7/1 -> Relational3/1
  Convert8/1 -> Relational3/2
  Relational3/1 -> Logical16/1
  Logical16/1 -> Logical9/2
  posedge2/1 -> Logical17/2
  Logical17/1 -> Logical2/2
  Inverter3/1 -> Logical17/1
  [valid2] -> Convert8/1
  [valid2] -> Convert4/1
  [valid2] -> Logical7/3
  [eof] -> Logical16/2
  [valid1] -> Logical4/2
  [valid1] -> Convert5/1
  [ok2] -> Logical10/2
  Inverter7/1 -> [ok2]
  Inverter6/1 -> [ok1]
  [ok1] -> Logical14/2
  [ok22] -> posedge3/1
  [ok22] -> Inverter3/1
  [valid1] -> Convert7/1
  Logical6/1 -> Counter6/4

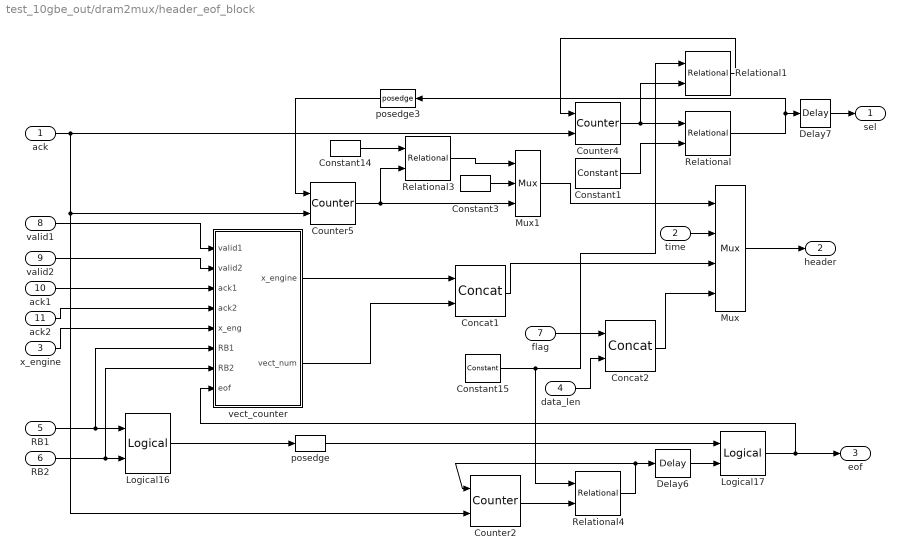
== system test_10gbe_out/dram2mux/header_eof_block ==
  ack : Inport  Port=1  LatchInput=off
  time : Inport  Port=2  LatchInput=off
  x_engine : Inport  Port=3  LatchInput=off
  data_len : Inport  Port=4  LatchInput=off
  RB1 : Inport  Port=5  LatchInput=off
  RB2 : Inport  Port=6  LatchInput=off
  flag : Inport  Port=7  LatchInput=off
  valid1 : Inport  Port=8  LatchInput=off
  valid2 : Inport  Port=9  LatchInput=off
  ack1 : Inport  Port=10  LatchInput=off
  ack2 : Inport  Port=11  LatchInput=off
  Concat1 : xbsIndex_r3/Concat  num_inputs=2  explicit_period=off  period=1  dbl_ovrd=off
  Concat2 : xbsIndex_r3/Concat  num_inputs=2  explicit_period=off  period=1  dbl_ovrd=off
  Constant1 : xbsIndex_r3/Constant  const=3  equ=P=C  arith_type=Unsigned  n_bits=16  bin_pt=0  opselect=C  inp2=PCIN>>17  opr=+  inp1=P  carry=CIN  iostate=0  explicit_period=on  period=1  dbl_ovrd=off
  Constant14 : xbsIndex_r3/Constant  const=2  equ=P=C  arith_type=Unsigned  n_bits=2  bin_pt=0  opselect=C  inp2=PCIN>>17  opr=+  inp1=P  carry=CIN  iostate=0  explicit_period=on  period=1  dbl_ovrd=off
  Constant15 : xbsIndex_r3/Constant  const=payload_len+3  equ=P=C  arith_type=Unsigned  n_bits=8  bin_pt=0  opselect=C  inp2=PCIN>>17  opr=+  inp1=P  carry=CIN  iostate=0  explicit_period=on  period=1  dbl_ovrd=off
  Constant3 : xbsIndex_r3/Constant  const=0  equ=P=C  arith_type=Unsigned  n_bits=1  bin_pt=0  opselect=C  inp2=PCIN>>17  opr=+  inp1=P  carry=CIN  iostate=0  explicit_period=on  period=1  dbl_ovrd=off
  Counter2 : xbsIndex_r3/Counter  cnt_type=Free Running  n_bits=32  bin_pt=0  arith_type=Unsigned  start_count=0  cnt_to=Inf  cnt_by_val=1  operation=Up  explicit_period=on  period=1  load_pin=off  rst=on  en=on  dbl_ovrd=off  show_param=off  use_rpm=on  gen_core=off
      settings: xl_area=[0, 0, 0, 0, 0, 0, 0]
  Counter4 : xbsIndex_r3/Counter  cnt_type=Free Running  n_bits=16  bin_pt=0  arith_type=Unsigned  start_count=0  cnt_to=Inf  cnt_by_val=1  operation=Up  explicit_period=on  period=1  load_pin=off  rst=on  en=on  dbl_ovrd=off  show_param=off  use_rpm=on  gen_core=off
      settings: xl_area=[0, 0, 0, 0, 0, 0, 0]
  Counter5 : xbsIndex_r3/Counter  cnt_type=Free Running  n_bits=2  bin_pt=0  arith_type=Unsigned  start_count=0  cnt_to=Inf  cnt_by_val=1  operation=Up  explicit_period=on  period=1  load_pin=off  rst=on  en=on  dbl_ovrd=off  show_param=off  use_rpm=on  gen_core=off
      settings: xl_area=[0, 0, 0, 0, 0, 0, 0]
  Delay6 : xbsIndex_r3/Delay  latency=1  reg_retiming=off  explicit_period=off  period=1  en=off  accept_only_valid=off  init_zero=on  dbl_ovrd=off  show_param=off
      settings: xl_area=[0, 0, 0, 0, 0, 0, 0]
  Delay7 : xbsIndex_r3/Delay  latency=1  reg_retiming=off  explicit_period=off  period=1  en=off  accept_only_valid=off  init_zero=on  dbl_ovrd=off  show_param=off
      settings: xl_area=[0, 0, 0, 0, 0, 0, 0]
  Logical16 : xbsIndex_r3/Logical  logical_function=OR  inputs=2  precision=Full  arith_type=Unsigned  n_bits=8  bin_pt=2  align_bp=on  latency=0  explicit_period=off  period=1  en=off  dbl_ovrd=off  show_param=off
      settings: xl_area=[0, 0, 0, 0, 0, 0, 0]
  Logical17 : xbsIndex_r3/Logical  logical_function=OR  inputs=2  precision=Full  arith_type=Unsigned  n_bits=8  bin_pt=2  align_bp=on  latency=0  explicit_period=off  period=1  en=off  dbl_ovrd=off  show_param=off
      settings: xl_area=[0, 0, 0, 0, 0, 0, 0]
  Mux : xbsIndex_r3/Mux  inputs=3  precision=Full  arith_type="Signed  (2's comp)"  n_bits=8  bin_pt=2  quantization=Truncate  overflow=Wrap  latency=2  explicit_period=on  period=1  en=off  dbl_ovrd=off  show_param=off  mux_type=off  use_rpm=off  gen_core=off
      settings: xl_area=[0, 0, 0, 0, 0, 0, 0]
  Mux1 : xbsIndex_r3/Mux  inputs=2  precision=Full  arith_type="Signed  (2's comp)"  n_bits=8  bin_pt=2  quantization=Truncate  overflow=Wrap  latency=0  explicit_period=off  period=1  en=off  dbl_ovrd=off  show_param=off  mux_type=off  use_rpm=off  gen_core=off
      settings: xl_area=[0, 0, 0, 0, 0, 0, 0]
  Relational : xbsIndex_r3/Relational  mode=a<b  latency=0  explicit_period=off  period=1  en=off  dbl_ovrd=off  show_param=off
      settings: xl_area=[0, 0, 0, 0, 0, 0, 0]
  Relational1 : xbsIndex_r3/Relational  mode=a=b  latency=0  explicit_period=off  period=1  en=off  dbl_ovrd=off  show_param=off
      settings: xl_area=[0, 0, 0, 0, 0, 0, 0]
  Relational3 : xbsIndex_r3/Relational  mode=a>=b  latency=0  explicit_period=off  period=1  en=off  dbl_ovrd=off  show_param=off
      settings: xl_area=[0, 0, 0, 0, 0, 0, 0]
  Relational4 : xbsIndex_r3/Relational  mode=a=b  latency=0  explicit_period=off  period=1  en=off  dbl_ovrd=off  show_param=off
      settings: xl_area=[0, 0, 0, 0, 0, 0, 0]
  posedge : casper_library/Misc/posedge  Tag=Rising Edge Detector
  posedge3 : casper_library/Misc/posedge  Tag=Rising Edge Detector  Orientation=left
  vect_counter : Subsystem
  sel : Outport
  header : Outport  Port=2
  eof : Outport  Port=3
  wires:
  Relational4/1 -> Counter2/1, Delay6/1
  Counter2/1 -> Relational4/2
  Relational1/1 -> Counter4/1
  Constant1/1 -> Relational/2
  Relational/1 -> posedge3/1, Delay7/1
  Counter4/1 -> Relational/1, Relational1/2
  flag/1 -> Concat2/1
  Concat1/1 -> Mux/3
  Concat2/1 -> Mux/4
  Constant15/1 -> Relational4/1, Relational1/1
  posedge3/1 -> Counter5/1
  Mux1/1 -> Mux/1
  Counter5/1 -> Mux1/3, Relational3/2
  Constant3/1 -> Mux1/2
  Constant14/1 -> Relational3/1
  Relational3/1 -> Mux1/1
  posedge/1 -> Logical17/1
  Delay6/1 -> Logical17/2
  Logical16/1 -> posedge/1
  ack/1 -> Counter4/2, Counter5/2, Counter2/2
  Delay7/1 -> sel/1
  time/1 -> Mux/2
  Mux/1 -> header/1
  data_len/1 -> Concat2/2
  RB1/1 -> Logical16/1, vect_counter/6(RB1)
  Logical17/1 -> eof/1, vect_counter/8(eof)
  RB2/1 -> Logical16/2, vect_counter/7(RB2)
  vect_counter/1(x_engine) -> Concat1/1
  vect_counter/2(vect_num) -> Concat1/2
  valid1/1 -> vect_counter/1(valid1)
  valid2/1 -> vect_counter/2(valid2)
  ack1/1 -> vect_counter/3(ack1)
  ack2/1 -> vect_counter/4(ack2)
  x_engine/1 -> vect_counter/5(x_eng)
